simulink model "MagnetoShield_PolePlacement_Simulation"  (R2019a)
settings: Solver=VariableStepAuto  StartTime=0.0  StopTime=24  RelTol=1e-3
values from neighbouring files (symbols this model uses):
  A = modeld.a    [LQR_initialization.m]    (also in LQ_observer_initialization.m; MPC_initialization.m = sysd.a; MagnetoShield_LQ_Initialization.m; MagnetoShield_PolePlacement_Initialization.m)
  B = modeld.b    [LQR_initialization.m]    (also in LQ_observer_initialization.m; MPC_initialization.m = sysd.b; MagnetoShield_LQ_Initialization.m; MagnetoShield_PolePlacement_Initialization.m)
  C = [1 0 0;0 0 1]    [LQR_initialization.m]    (also in LQ_observer_initialization.m = [1 0 0]; MPC_initialization.m = [1 0 0]; MagnetoShield_LQ_Initialization.m; MagnetoShield_PolePlacement_Initialization.m = [1 0 0])
  i0 = 0.00301720799779    [MagnetoShield_Alternative_model.mat]    (also in MagnetoShield_Models_Greybox_SS model.mat = 0.0219057293333)
  K = dlqr(Ai,Bi,Qlq,Rlq)    [LQR_initialization.m]    (also in LQ_observer_initialization.m; MagnetoShield_LQ_Initialization.m; MagnetoShield_PolePlacement_Initialization.m = [0 0 0 1]*inv([Bi Ai*Bi Ai^2*Bi Ai^3*Bi])*phy)
  L = phy*inv([C; C*A; C*A^2])*[0 0 1]'    [LQ_observer_initialization.m]    (also in MagnetoShield_PolePlacement_Initialization.m)
  Ts = 0.001    [LQR_initialization.m]    (also in LQ_observer_initialization.m = 0.002; MPC_initialization.m; MagnetoShield_LQ_Initialization.m = 0.0015; MagnetoShield_PolePlacement_Initialization.m = 0.0015)
  u0 = 0.633613679536    [MagnetoShield_Alternative_model.mat]    (also in MagnetoShield_Models_Greybox_SS model.mat = 4.62338933333)
  y0 = 0.012    [MagnetoShield_Alternative_model.mat]    (also in MagnetoShield_Models_Greybox_SS model.mat = 0.0143094466667)
undefined symbols (not defined in the file or in its folder): DiscIntNeverNeededParam
libraries: simulink x2
settings Model: Creator=jakub  LastModifiedBy=jakub
settings SolverCC: AlgebraicLoopSolver=LineSearch

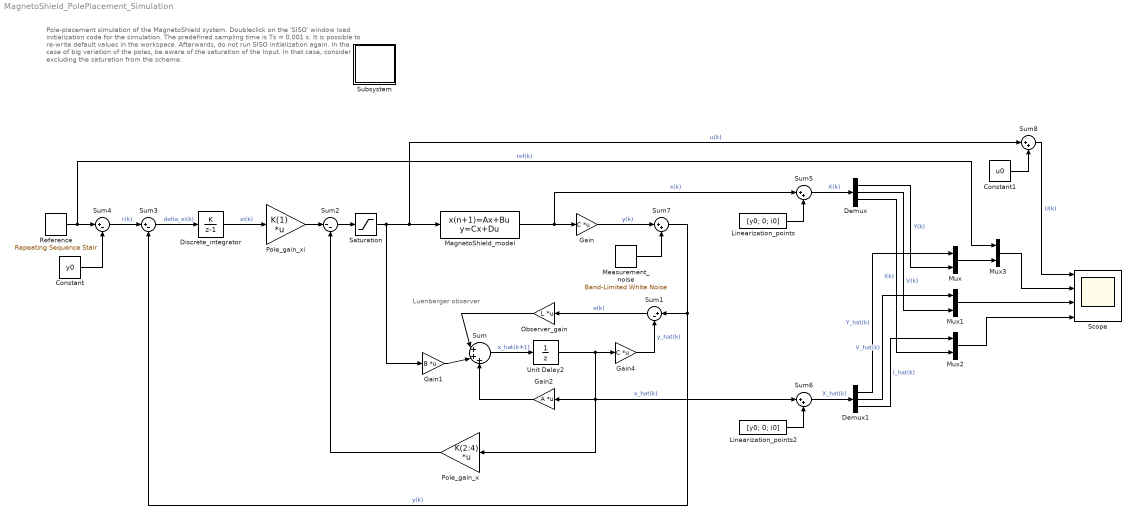
== system MagnetoShield_PolePlacement_Simulation ==
  note: Luenberger observer
  note: Pole-placement simulation of the MagnetoShield system.
      | Doubleclick on the 'SISO' window load initialization code for the simulation.
      | The predefined sampling time is Ts = 0.001 s. It is possible to re-write default values in the
      | workspace. Afterwards, do not run SISO initialization again.
      |
      | In the case of big variation of the poles, be aware of the saturation of the Input. In that case,
      | consider excluding the saturation from the scheme.
  Constant : Constant  Value=y0
  Constant1 : Constant  Value=u0
  Demux : Demux  Outputs=3
  Demux1 : Demux  Outputs=3
  Discrete_integrator : DiscreteIntegrator  IntegratorMethod=Accumulation: Forward Euler  SampleTime=Ts  LimitOutput=on  UpperSaturationLimit=1  LowerSaturationLimit=-1  ICPrevOutput=DiscIntNeverNeededParam  ICPrevScaledInput=DiscIntNeverNeededParam
  Gain : Gain  Gain=C  Multiplication=Matrix(K*u)
  Gain1 : Gain  Gain=B  Multiplication=Matrix(K*u)
  Gain2 : Gain  Gain=A  Multiplication=Matrix(K*u)
  Gain4 : Gain  Gain=C  Multiplication=Matrix(K*u)
  Linearization_points : Constant  Value=[y0; 0; i0]
  Linearization_points2 : Constant  Value=[y0; 0; i0]
  MagnetoShield_model : DiscreteStateSpace  A=A  B=B  C=[1 0 0;0 1 0;0 0 1]  D=[0;0;0]  InitialCondition=[0.017-y0;0;0-i0]  SampleTime=Ts
  Measurement_noise : simulink/Sources/Band-Limited White Noise  Cov=[(2*10^(-8))^2]  Ts=2*Ts  seed=[23341]
  Mux{,1..3} (4 alike) : Mux  Inputs=2
  Observer_gain : Gain  Gain=L  Multiplication=Matrix(K*u)
  Pole_gain_x : Gain  Gain=K(2:4)  Multiplication=Matrix(K*u)
  Pole_gain_xi : Gain  Gain=K(1)  Multiplication=Matrix(K*u)
  Reference : simulink/Sources/Repeating Sequence Stair  OutValues=[ones(1,2000)*0.013 ones(1,2000)*0.016 ones(1,2000)*0.012].'  tsamp=Ts  OutMin=[]  OutMax=[]  OutDataTypeStr=double  OutputDataTypeScalingMode=double  OutDataType=fixdt(0,8)  ConRadixGroup=Best Precision: Vector-wise  OutScaling=2^-12
  Saturation : Saturate  UpperLimit=12-u0  LowerLimit=0-u0
  Scope : Scope  NumInputPorts=4
  Subsystem : Subsystem
      settings: OpenFcn=|
      | clear;close all;clc;
      | cd(fileparts(which(gcs)));
      | load '../../../matlab/examples/MagnetoShield/MagnetoShield_Models_Greybox_SS';
      | %% MagnetoShield - Pole-placement simulation and control initialization for Simulink
      | Ts = 0.001;                   % Sampling of the Simulink simulation
      | 
      | % Matrices extraction from model
      | modeld=c2d(model,Ts);           % Discretized linear state-space model
      | A = modeld.a;                   % Extract A
      | B = modeld.b;                   % Extract B
      | C = [1 0 0];                   % Position is measured for integrator 'xi' computation
      | 
      | % Discrete augmented model with integrator state - unstable, unobservable
      | Ai = [1 -C;
      |       zeros(3,1) A];
      | Bi = [0;B];
      | 
      | % Observer gain L computation
      | polesL = [-0.003 0.0006715 -0.00003715]; % desired poles of observer
      | p = poly(polesL);                        % polynomial coeficients
      | I = eye(size(A));
      | phy = p(4)*I+p(3)*A+p(2)*A^2+A^3;
      | L = phy*inv([C; C*A; C*A^2])*[0 0 1]';   % Ackermann's formula for observer
      | 
      | % Pole-placement gain K for augmented system
      | polesK = [0.985 0.5353 0.826 0.9581];       % desired poles of the system
      | p = poly(polesK);                           % polynomial coeficients
      | I = eye(size(Ai));
      | phy = p(5)*I+p(4)*Ai+p(3)*Ai^2+p(2)*Ai^3+Ai^4;
      | K = [0 0 0 1]*inv([Bi Ai*Bi Ai^2*Bi Ai^3*Bi])*phy; % Ackermann's formula for gain K
      mask Display: disp('SISO')
  Sum : Sum  Inputs=|+++
  Sum1 : Sum  Inputs=|+-
  Sum2 : Sum  Inputs=|--
  Sum3 : Sum  Inputs=|+-
  Sum4 : Sum  Inputs=|+-
  Sum{5..8} (4 alike) : Sum  Inputs=|++
  Unit Delay2 : UnitDelay  InitialCondition=[0.017-y0;0;0-i0]  SampleTime=-1  HasFrameUpgradeWarning=on
  wires:
  Saturation/1 -> Sum8/1, MagnetoShield_model/1, Gain1/1  "u(k)"
  Sum2/1 -> Saturation/1
  Discrete_integrator/1 -> Pole_gain_xi/1  "xi(k)"
  Sum3/1 -> Discrete_integrator/1  "delta_xi(k)"
  Pole_gain_xi/1 -> Sum2/1
  Reference/1 -> Mux3/1, Sum4/1  "ref(k)"
  Pole_gain_x/1 -> Sum2/2
  MagnetoShield_model/1 -> Sum5/1, Gain/1  "x(k)"
  Gain1/1 -> Sum/2
  Unit Delay2/1 -> Gain4/1, Pole_gain_x/1, Gain2/1, Sum6/1  "x_hat(k)"
  Gain2/1 -> Sum/3
  Sum1/1 -> Observer_gain/1  "e(k)"
  Gain4/1 -> Sum1/2  "y_hat(k)"
  Observer_gain/1 -> Sum/1
  Sum/1 -> Unit Delay2/1  "x_hat(k+1)"
  Sum7/1 -> Sum3/2, Sum1/1  "y(k)"
  Measurement_noise/1 -> Sum7/2
  Gain/1 -> Sum7/1  "y(k)"
  Mux/1 -> Mux3/2
  Mux1/1 -> Scope/3
  Mux2/1 -> Scope/4
  Demux/1 -> Mux/2  "Y(k)"
  Demux1/1 -> Mux/1  "Y_hat(k)"
  Demux/2 -> Mux1/2  "V(k)"
  Demux1/2 -> Mux1/1  "V_hat(k)"
  Demux1/3 -> Mux2/1  "I_hat(k)"
  Demux/3 -> Mux2/2  "I(k)"
  Sum4/1 -> Sum3/1  "r(k)"
  Constant/1 -> Sum4/2
  Sum5/1 -> Demux/1  "X(k)"
  Sum6/1 -> Demux1/1  "X_hat(k)"
  Linearization_points/1 -> Sum5/2
  Linearization_points2/1 -> Sum6/2
  Constant1/1 -> Sum8/2
  Sum8/1 -> Scope/1  "U(k)"
  Mux3/1 -> Scope/2

== system MagnetoShield_PolePlacement_Simulation/Subsystem ==
